simulink model "Forword"  (Simulink 6.1)
settings: Solver=ode23tb  StartTime=0.0  StopTime=0.003  MaxStep=1e-6  RelTol=1e-3  AbsTol=.01
libraries: powerlib x11
settings Model: LastModifiedBy=ThinkPad
settings DebuggingCC: SolverPrmCheckMsg=warning

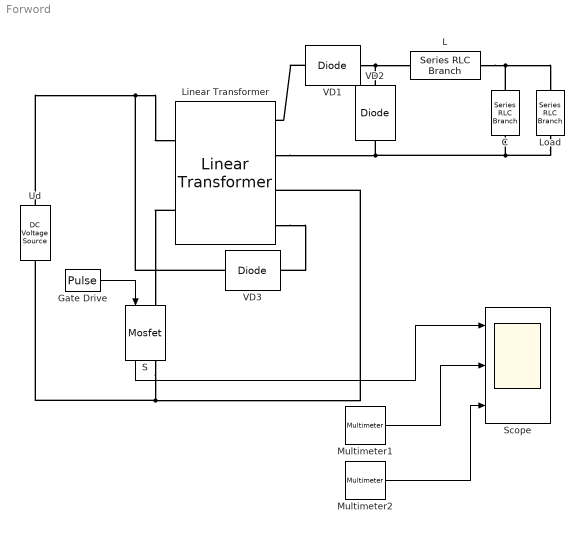
== system Forword ==
  C : powerlib/Elements/Series RLC Branch  Orientation=up  PhysicalDomain=powersysdomain  SubClassName=unknown  LeftPortType=p1  RightPortType=p1  LConnTagsString=__new0  RConnTagsString=__new0  Resistance=0  Inductance=0  Capacitance=50e-6  Measurements=None
  Gate Drive : DiscretePulseGenerator  PulseType=Time based  Period=0.00005  PulseWidth=40
  L : powerlib/Elements/Series RLC Branch  PhysicalDomain=powersysdomain  SubClassName=unknown  LeftPortType=p1  RightPortType=p1  LConnTagsString=__new0  RConnTagsString=__new0  Resistance=0  Inductance=0.001  Capacitance=inf  Measurements=Branch current
  Linear Transformer : powerlib/Elements/Linear Transformer  PhysicalDomain=powersysdomain  SubClassName=unknown  LeftPortType=p1  RightPortType=p1  LConnTagsString=a|b  RConnTagsString=A|B|C|D  NominalPower=[1000 20e3 ]  winding1="[ 100  0.002  0.001 ]"  winding2="[ 100  0.002  0.001 ]"  ThreeWindings=on  winding3=[ 100 0.005 0.001 ]  RmLm=[ 100 20 ]  Measurements=Magnetization current
  Load : powerlib/Elements/Series RLC Branch  Orientation=down  PhysicalDomain=powersysdomain  SubClassName=unknown  LeftPortType=p1  RightPortType=p1  LConnTagsString=__new0  RConnTagsString=__new0  Resistance=4  Inductance=0  Capacitance=inf  Measurements=Branch voltage
  Multimeter1 : powerlib/Measurements/Multimeter  PhasorSimulation=off  OutputType=Complex  sel=[2 3]  L=3  Gain=[1 1]  yselected={'Ib: L','Imag: Linear Transformer'};  PSBOutputType=1  PSBequivalent=0  AxesSetting=[0,0.1,-100,100]  Display=0  SavedBlockNames=-11
  Multimeter2 : powerlib/Measurements/Multimeter  PhasorSimulation=off  OutputType=Complex  sel=1  L=3  Gain=1  yselected={'Ub: Load'};  PSBOutputType=1  PSBequivalent=0  AxesSetting=[0,0.1,-100,100]  Display=0  SavedBlockNames=-11
  S : powerlib/Power Electronics/Mosfet  Orientation=down  Ron=0.01  Lon=1e-9  Rd=.01  IC=0  Rs=10  Cs=1e-9  Measurements=on
  Scope : Scope  NumInputPorts=3
      settings: TimeRange=0.0005  YMin=-50~-5~0  YMax=250~20~60  SampleTime=2e-4
  Ud : powerlib/Electrical Sources/DC Voltage Source  Orientation=up  Amplitude=100  Measurements=None
  VD1 : powerlib/Power Electronics/Diode  Ron=0.001  Lon=0  Vf=0  IC=0  Rs=10  Cs=1e-9  Measurements=off
  VD2 : powerlib/Power Electronics/Diode  Orientation=up  Ron=0.001  Lon=0  Vf=0  IC=0  Rs=10  Cs=1e-9  Measurements=off
  VD3 : powerlib/Power Electronics/Diode  Orientation=left  Ron=0.001  Lon=0  Vf=0.8  IC=0  Rs=10  Cs=1e-9  Measurements=off
  wires:
  Gate Drive/1 -> S/1
  S/1 -> Scope/1
  Multimeter1/1 -> Scope/2
  Multimeter2/1 -> Scope/3
  connections:
  Linear Transformer/RConn3 -- S/RConn1 -- Ud/LConn1
  Linear Transformer/LConn2 -- S/LConn1
  Ud/RConn1 -- Linear Transformer/LConn1 -- VD3/RConn1
  Load/RConn1 -- Linear Transformer/RConn2 -- VD2/LConn1 -- C/LConn1
  C/RConn1 -- Load/LConn1 -- L/RConn1
  Linear Transformer/RConn4 -- VD3/LConn1
  VD2/RConn1 -- L/LConn1 -- VD1/RConn1
  VD1/LConn1 -- Linear Transformer/RConn1
